simulink subsystem "Executive"  (R2025b)
settings: Solver=VariableStepAuto  StartTime=0.0  StopTime=10.0  RelTol=1e-3
undefined symbols (not defined in the file or in its folder): dt_control
settings Model: Creator=kjhaydon  LastModifiedBy=koryh

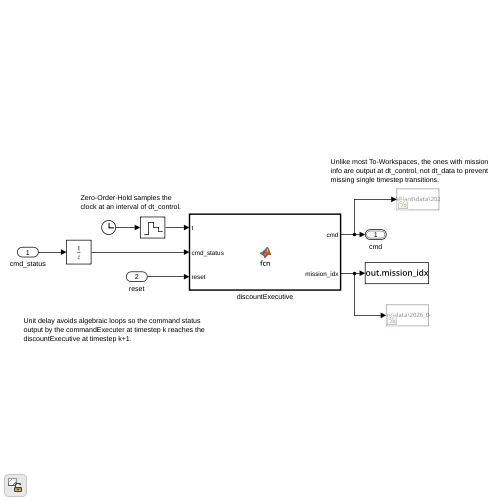
[thumbnail: Simulink's stored preview of the top-level diagram]
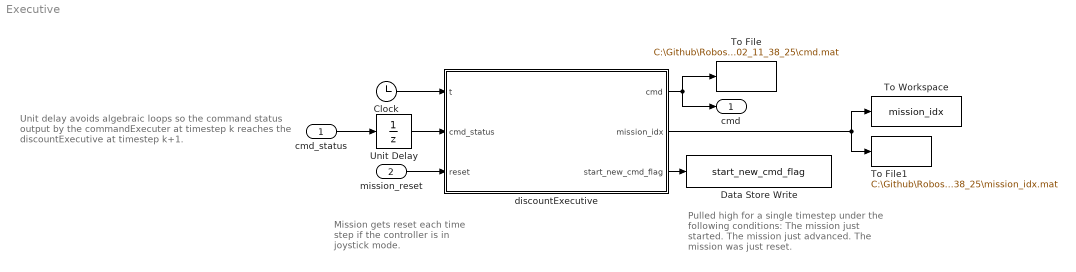
== system Executive ==
  note: Pulled high for a single timestep under the following conditions:
      | The mission just started.
      | The mission just advanced.
      | The mission was just reset.
  note: Unit delay avoids algebraic loops so the command status
      | output by the commandExecuter at timestep k reaches the
      | discountExecutive at timestep k+1.
  note: Mission gets reset each time step if the controller is in joystick mode.
  cmd_status : Inport  SampleTime=dt_control
  mission_reset : Inport  Port=2
  Clock : Clock
  Data Store Write : DataStoreWrite  DataStoreName=start_new_cmd_flag  IndexOptions=Index vector (dialog)  Indices=1  OutputSizes=1
  To File : ToFile  Filename=C:\Github\Robosub\SimulinkPlant\data\2026_05_02_11_38_25\cmd.mat  MatrixName=cmd  SaveFormat=Timeseries
  To File1 : ToFile  Filename=C:\Github\Robosub\SimulinkPlant\data\2026_05_02_11_38_25\mission_idx.mat  MatrixName=mission_idx  SaveFormat=Timeseries
  To Workspace : ToWorkspace  VariableName=mission_idx  SaveFormat=Timeseries  SampleTime=dt_control
  Unit Delay : UnitDelay  InitialCondition=int8('RUNN')'  SampleTime=-1  HasFrameUpgradeWarning=on
  discountExecutive : MATLAB Function  TreatAsAtomicUnit=on
  cmd : Outport  OutDataTypeStr=Bus: cmd_bus
      settings: VarSizeSig=Yes
  wires:
  Unit Delay/1 -> discountExecutive/2(cmd_status)
  cmd_status/1 -> Unit Delay/1
  Clock/1 -> discountExecutive/1(t)
  mission_reset/1 -> discountExecutive/3(reset)
  discountExecutive/2(mission_idx) -> To Workspace/1, To File1/1
  discountExecutive/1(cmd) -> To File/1, cmd/1
  discountExecutive/3(start_new_cmd_flag) -> Data Store Write/1

== matlab function Executive/discountExecutive ==
  settings: updateMethod=DISCRETE  sampleTime=dt_control
  data: t input; cmd_status input; cmd output Bus: cmd_bus; mission parameter Bus: cmd_bus size=max_commands_in_mission; mission_idx output; reset input boolean; start_new_cmd_flag output
function [cmd, mission_idx, start_new_cmd_flag] = fcn(t, cmd_status, mission, reset)

[cmd, mission_idx, start_new_cmd_flag] = discountExecutive(t, cmd_status, mission, reset);
